simulink subsystem "execute_command"  (R2025b)
settings: Solver=VariableStepAuto  StartTime=0.0  StopTime=10.0  RelTol=1e-3
undefined symbols (not defined in the file or in its folder): dt_control, dt_data
settings Model: Creator=kjhaydon  LastModifiedBy=kjhaydon

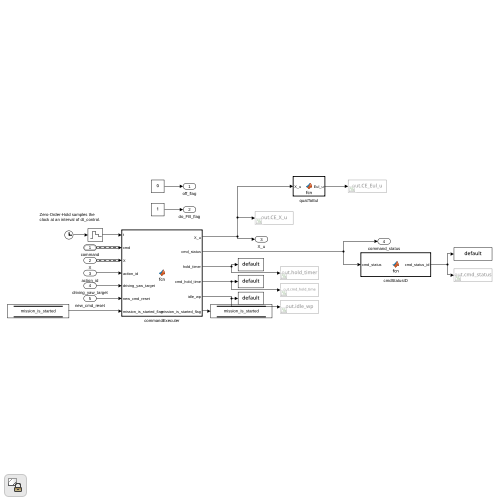
[thumbnail: Simulink's stored preview of the top-level diagram]
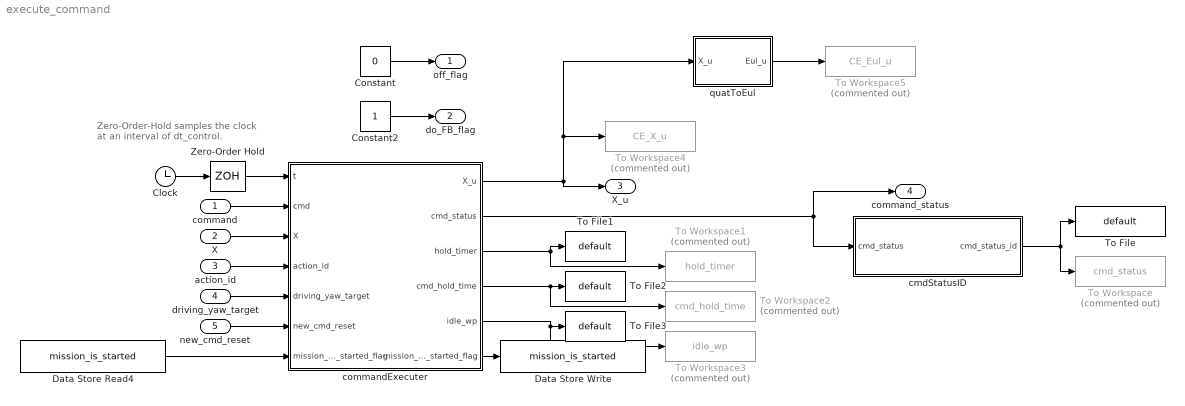
== system execute_command ==
  note: Zero-Order-Hold samples the
      | clock at an interval of dt_control.
  command : Inport  OutDataTypeStr=Bus: cmd_bus  SampleTime=dt_control
  X : Inport  Port=2  SampleTime=dt_control
  action_id : Inport  Port=3  SampleTime=dt_control
  driving_yaw_target : Inport  Port=4  SampleTime=dt_control
  new_cmd_reset : Inport  Port=5  SampleTime=dt_control
  Clock : Clock
  Constant : Constant  Value=0
  Constant2 : Constant
  Data Store Read4 : DataStoreRead  DataStoreName=mission_is_started  IndexOptions=Index vector (dialog)  Indices=1  OutputSizes=1
  Data Store Write : DataStoreWrite  DataStoreName=mission_is_started  IndexOptions=Index vector (dialog)  Indices=1  OutputSizes=1
  To File : ToFile  Filename=default  MatrixName=cmd_status  SaveFormat=Timeseries
  To File1 : ToFile  Filename=default  MatrixName=hold_timer  SaveFormat=Timeseries
  To File2 : ToFile  Filename=default  MatrixName=cmd_hold_time  SaveFormat=Timeseries
  To File3 : ToFile  Filename=default  MatrixName=idle_wp  SaveFormat=Timeseries
  To Workspace : ToWorkspace  Commented=on  VariableName=cmd_status  SaveFormat=Timeseries  SampleTime=dt_control
  To Workspace1 : ToWorkspace  Commented=on  VariableName=hold_timer  SaveFormat=Timeseries  SampleTime=dt_control
  To Workspace2 : ToWorkspace  Commented=on  VariableName=cmd_hold_time  SaveFormat=Timeseries  SampleTime=dt_control
  To Workspace3 : ToWorkspace  Commented=on  VariableName=idle_wp  SaveFormat=Timeseries  SampleTime=dt_control
  To Workspace4 : ToWorkspace  Commented=on  VariableName=CE_X_u  SaveFormat=Timeseries  SampleTime=dt_data
  To Workspace5 : ToWorkspace  Commented=on  VariableName=CE_Eul_u  SaveFormat=Timeseries  SampleTime=dt_data
  Zero-Order Hold : ZeroOrderHold  SampleTime=dt_control
  cmdStatusID : MATLAB Function  TreatAsAtomicUnit=on
  commandExecuter : MATLAB Function  TreatAsAtomicUnit=on
  quatToEul : MATLAB Function  TreatAsAtomicUnit=on
  off_flag : Outport
  do_FB_flag : Outport  Port=2
  X_u : Outport  Port=3
  command_status : Outport  Port=4
  wires:
  Constant/1 -> off_flag/1
  Constant2/1 -> do_FB_flag/1
  commandExecuter/1(X_u) -> quatToEul/1(X_u), To Workspace4/1, X_u/1
  commandExecuter/2(cmd_status) -> command_status/1, cmdStatusID/1(cmd_status)
  cmdStatusID/1(cmd_status_id) -> To Workspace/1, To File/1
  commandExecuter/3(hold_timer) -> To File1/1, To Workspace1/1
  commandExecuter/4(cmd_hold_time) -> To File2/1, To Workspace2/1
  Clock/1 -> Zero-Order Hold/1
  commandExecuter/5(idle_wp) -> To File3/1, To Workspace3/1
  quatToEul/1(Eul_u) -> To Workspace5/1
  new_cmd_reset/1 -> commandExecuter/6(new_cmd_reset)
  action_id/1 -> commandExecuter/4(action_id)
  driving_yaw_target/1 -> commandExecuter/5(driving_yaw_target)
  command/1 -> commandExecuter/2(cmd)
  X/1 -> commandExecuter/3(X)
  Zero-Order Hold/1 -> commandExecuter/1(t)
  Data Store Read4/1 -> commandExecuter/7("mission_is_started_flag ")
  commandExecuter/6(mission_is_started_flag) -> Data Store Write/1

== matlab function execute_command/cmdStatusID ==
  settings: updateMethod=DISCRETE  sampleTime=dt_control
  data: cmd_status_id output; cmd_status input
function cmd_status_id = fcn(cmd_status)

cmd_status_id = cmdStatusID(cmd_status);

== matlab function execute_command/commandExecuter ==
  settings: updateMethod=DISCRETE  sampleTime=dt_control
  data: X_u output size=[13 1]; cmd_status output int8 size=[4 1]; hold_timer output; cmd_hold_time output; idle_wp output; t input; cmd input; X input; action_id input; driving_yaw_target input; new_cmd_reset input; mission_is_started_flag input; mission_is_started_flag output
function [X_u, cmd_status, hold_timer, cmd_hold_time, idle_wp, mission_is_started_flag]  = fcn(t, cmd, X, action_id, driving_yaw_target,new_cmd_reset, mission_is_started_flag)

[X_u, cmd_status, hold_timer, cmd_hold_time, idle_wp, mission_is_started_flag] = commandExecuter(t, cmd, X, action_id, driving_yaw_target,new_cmd_reset, mission_is_started_flag);

== matlab function execute_command/quatToEul ==
  data: X_u input; Eul_u output
function Eul_u = fcn(X_u)

qib_u = X_u(4:7);

Eul_u = quatToEul(qib_u);
